simulink model "lista1_questao4"  (R2014b)
settings: Solver=ode45  StartTime=0.0  StopTime=60  RelTol=1e-3
libraries: cstblocks x1
settings Model: Creator=Danilo  LastModifiedBy=Danilo

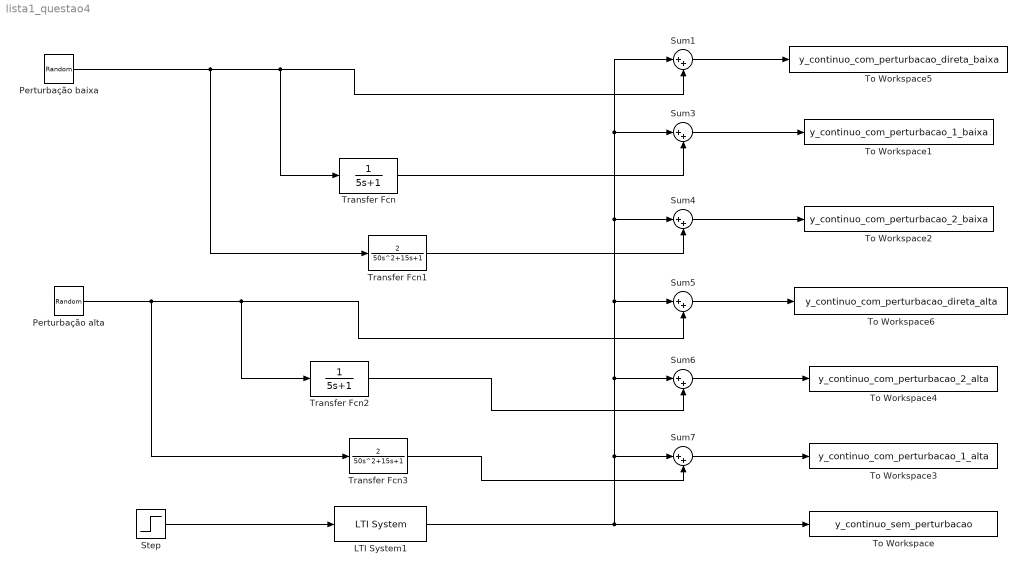
== system lista1_questao4 ==
  LTI System1 : cstblocks/LTI System  sys=H  IC=[]
  "Perturbação alta " : RandomNumber  Variance=0.1  SampleTime=0.1
  Perturbação baixa : RandomNumber  Variance=0.001  SampleTime=0.1
  Step : Step  Before=0.1  SampleTime=0
  Sum{1,3..7} (6 alike) : Sum  Inputs=|++
  To Workspace : ToWorkspace  VariableName=y_continuo_sem_perturbacao  SaveFormat=Timeseries  SampleTime=-1
  To Workspace1 : ToWorkspace  VariableName=y_continuo_com_perturbacao_1_baixa  SaveFormat=Timeseries  SampleTime=-1
  To Workspace2 : ToWorkspace  VariableName=y_continuo_com_perturbacao_2_baixa  SaveFormat=Timeseries  SampleTime=-1
  To Workspace3 : ToWorkspace  VariableName=y_continuo_com_perturbacao_1_alta  SaveFormat=Timeseries  SampleTime=-1
  To Workspace4 : ToWorkspace  VariableName=y_continuo_com_perturbacao_2_alta  SaveFormat=Timeseries  SampleTime=-1
  To Workspace5 : ToWorkspace  VariableName=y_continuo_com_perturbacao_direta_baixa  SaveFormat=Timeseries  SampleTime=-1
  To Workspace6 : ToWorkspace  VariableName=y_continuo_com_perturbacao_direta_alta  SaveFormat=Timeseries  SampleTime=-1
  Transfer Fcn : TransferFcn  Denominator=[5 1]
  Transfer Fcn1 : TransferFcn  Numerator=[2]  Denominator=[50 15 1]
  Transfer Fcn2 : TransferFcn  Denominator=[5 1]
  Transfer Fcn3 : TransferFcn  Numerator=[2]  Denominator=[50 15 1]
  wires:
  Step/1 -> LTI System1/1
  LTI System1/1 -> Sum7/1, Sum6/1, Sum5/1, Sum4/1, Sum3/1, Sum1/1, To Workspace/1
  Sum3/1 -> To Workspace1/1
  Sum1/1 -> To Workspace5/1
  Sum4/1 -> To Workspace2/1
  Sum5/1 -> To Workspace6/1
  Sum6/1 -> To Workspace4/1
  Sum7/1 -> To Workspace3/1
  "Perturbação alta "/1 -> Transfer Fcn3/1, Sum5/2, Transfer Fcn2/1
  Transfer Fcn/1 -> Sum3/2
  Transfer Fcn1/1 -> Sum4/2
  Transfer Fcn2/1 -> Sum6/2
  Transfer Fcn3/1 -> Sum7/2
  Perturbação baixa/1 -> Transfer Fcn1/1, Sum1/2, Transfer Fcn/1
